simulink model "a2_df1_mdl"  (R2020a)
settings: Solver=VariableStepAuto  StartTime=0.0  StopTime=10.0  RelTol=1e-3
settings Model: Creator=soymarwin  LastModifiedBy=soymarwin

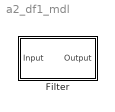
== system a2_df1_mdl ==
  Filter : Subsystem  Tag=FilterWizardSubSystem
      settings: ErrorFcn=dspFilterRealizedInBasicElemsAlgLoopErrFcnCallback

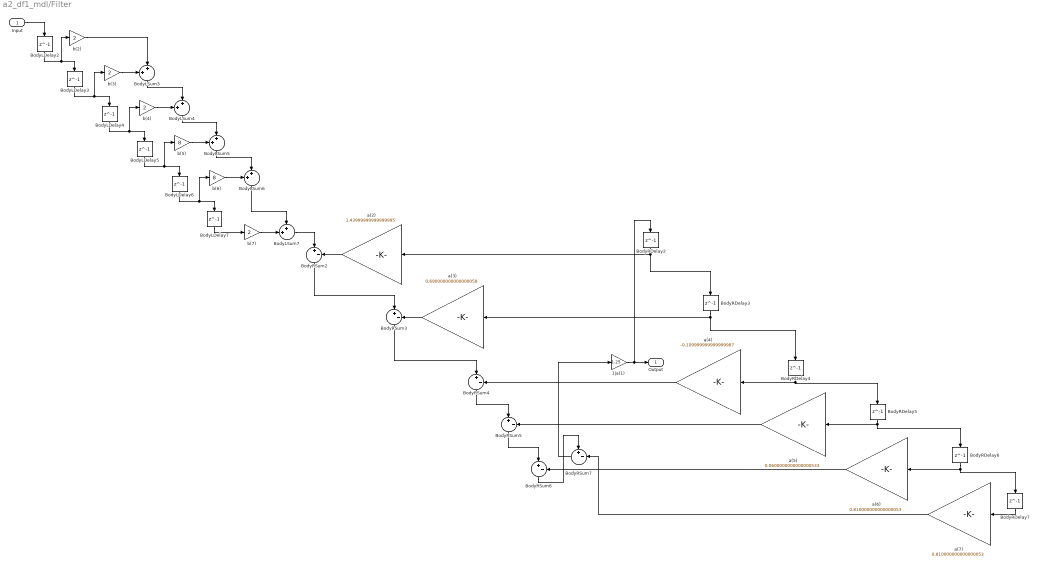
== system a2_df1_mdl/Filter ==
  Input : Inport
  1|a(1) : Gain  Gain=1.25  ParamDataTypeStr=double  RndMeth=Nearest  SaturateOnIntegerOverflow=on  OutDataTypeStr=Inherit: Same as input
  BodyLDelay{2..7} (6 alike) : Delay  DelayLength=1  InitialCondition=0
  BodyLSum{3..7} (5 alike) : Sum  Inputs=++|  RndMeth=Nearest  SaturateOnIntegerOverflow=on  OutDataTypeStr=Inherit: Same as first input
  BodyRDelay{2..7} (6 alike) : Delay  DelayLength=1  InitialCondition=0
  BodyRSum{2..6} (5 alike) : Sum  Inputs=|+-  RndMeth=Nearest  SaturateOnIntegerOverflow=on  OutDataTypeStr=Inherit: Same as first input
  BodyRSum7 : Sum  Inputs=+-|  RndMeth=Nearest  SaturateOnIntegerOverflow=on  OutDataTypeStr=Inherit: Same as first input
  a(2) : Gain  Gain=1.43999999999999995  ParamDataTypeStr=double  RndMeth=Nearest  SaturateOnIntegerOverflow=on  OutDataTypeStr=Inherit: Same as input
  a(3) : Gain  Gain=0.690000000000000058  ParamDataTypeStr=double  RndMeth=Nearest  SaturateOnIntegerOverflow=on  OutDataTypeStr=Inherit: Same as input
  a(4) : Gain  Gain=-0.109999999999999987  ParamDataTypeStr=double  RndMeth=Nearest  SaturateOnIntegerOverflow=on  OutDataTypeStr=Inherit: Same as input
  a(5) : Gain  Gain=0.0600000000000000533  ParamDataTypeStr=double  RndMeth=Nearest  SaturateOnIntegerOverflow=on  OutDataTypeStr=Inherit: Same as input
  a(6) : Gain  Gain=0.810000000000000053  ParamDataTypeStr=double  RndMeth=Nearest  SaturateOnIntegerOverflow=on  OutDataTypeStr=Inherit: Same as input
  a(7) : Gain  Gain=0.810000000000000053  ParamDataTypeStr=double  RndMeth=Nearest  SaturateOnIntegerOverflow=on  OutDataTypeStr=Inherit: Same as input
  b(2) : Gain  Gain=2  ParamDataTypeStr=double  RndMeth=Nearest  SaturateOnIntegerOverflow=on  OutDataTypeStr=Inherit: Same as input
  b(3) : Gain  Gain=2  ParamDataTypeStr=double  RndMeth=Nearest  SaturateOnIntegerOverflow=on  OutDataTypeStr=Inherit: Same as input
  b(4) : Gain  Gain=2  ParamDataTypeStr=double  RndMeth=Nearest  SaturateOnIntegerOverflow=on  OutDataTypeStr=Inherit: Same as input
  b(5) : Gain  Gain=8  ParamDataTypeStr=double  RndMeth=Nearest  SaturateOnIntegerOverflow=on  OutDataTypeStr=Inherit: Same as input
  b(6) : Gain  Gain=8  ParamDataTypeStr=double  RndMeth=Nearest  SaturateOnIntegerOverflow=on  OutDataTypeStr=Inherit: Same as input
  b(7) : Gain  Gain=2  ParamDataTypeStr=double  RndMeth=Nearest  SaturateOnIntegerOverflow=on  OutDataTypeStr=Inherit: Same as input
  Output : Outport
  wires:
  a(7)/1 -> BodyRSum7/2
  BodyRSum6/1 -> BodyRSum7/1
  BodyRDelay7/1 -> a(7)/1
  b(7)/1 -> BodyLSum7/2
  BodyRSum7/1 -> 1|a(1)/1
  BodyLDelay7/1 -> b(7)/1
  a(2)/1 -> BodyRSum2/2
  BodyLSum7/1 -> BodyRSum2/1
  BodyRDelay2/1 -> a(2)/1, BodyRDelay3/1
  BodyLDelay3/1 -> b(3)/1, BodyLDelay4/1
  a(6)/1 -> BodyRSum6/2
  BodyLSum6/1 -> BodyLSum7/1
  b(6)/1 -> BodyLSum6/1
  a(5)/1 -> BodyRSum5/2
  BodyRSum5/1 -> BodyRSum6/1
  BodyLSum5/1 -> BodyLSum6/2
  b(5)/1 -> BodyLSum5/1
  a(4)/1 -> BodyRSum4/2
  BodyRSum4/1 -> BodyRSum5/1
  BodyLSum4/1 -> BodyLSum5/2
  b(4)/1 -> BodyLSum4/1
  BodyRDelay3/1 -> a(3)/1, BodyRDelay4/1
  a(3)/1 -> BodyRSum3/2
  BodyRDelay6/1 -> a(6)/1, BodyRDelay7/1
  BodyLSum3/1 -> BodyLSum4/2
  BodyRSum3/1 -> BodyRSum4/1
  b(3)/1 -> BodyLSum3/1
  BodyRSum2/1 -> BodyRSum3/1
  b(2)/1 -> BodyLSum3/2
  BodyLDelay5/1 -> b(5)/1, BodyLDelay6/1
  Input/1 -> BodyLDelay2/1
  BodyLDelay6/1 -> b(6)/1, BodyLDelay7/1
  BodyRDelay5/1 -> a(5)/1, BodyRDelay6/1
  BodyRDelay4/1 -> a(4)/1, BodyRDelay5/1
  BodyLDelay4/1 -> b(4)/1, BodyLDelay5/1
  BodyLDelay2/1 -> b(2)/1, BodyLDelay3/1
  1|a(1)/1 -> Output/1, BodyRDelay2/1
